simulink model "motor_model"  (R2026a)
settings: Solver=VariableStepAuto  StopTime=30  FixedStep=-1
model workspace (MAT data in the model file):
  g = 9.81
  k = 2
  r = 0.05
  t = 1800
  zs = [1.77 0.0139]
values from neighbouring files (symbols this model uses):
  amb_temp = 25    [datagenerationcode.m]
  current_gain = 1.0    (= 1)    [datagenerationcode.m]
  fault_enable = (fault_mask ~= 0)    [datagenerationcode.m]
  fault_mask = fault_masks(m)    [datagenerationcode.m]
  temp_gain = 1.0    (= 1)    [datagenerationcode.m]
  ts = 0.02    [datagenerationcode.m]
  vib_gain = 1.0    (= 1)    [datagenerationcode.m]
libraries: simulink x8, fl_lib x6, nesl_utility x3, dspfdesign x1, autolibim x1
settings Model: Creator=Onabanjo Daniel
settings SimscapeCC: SimscapeNominalValues="[{\"value\":\"1\",\"unit\":\"A\"},{\"value\":\"1\",\"unit\":\"bar\"},{\"value\":\"1\",\"unit\":\"cm^2\"},{\"value\":\"1\",\"unit\":\"cm^3/s\"},{\"value\":\"1\",\"unit\":\"kJ/kg\"},{\"value\":\"1\",\"unit\":\"kW\"},{\"value\":\"1\",\"unit\":\"l\"},{\"value\":\"1\",\"unit\":\"N\"},{\"value\":\"1\",\"unit\":\"N*m\"},{\"value\":\"1\",\"unit\":\"V\"}]"  SimscapeLogType=none  SimscapeLogDataHistory=5000.0

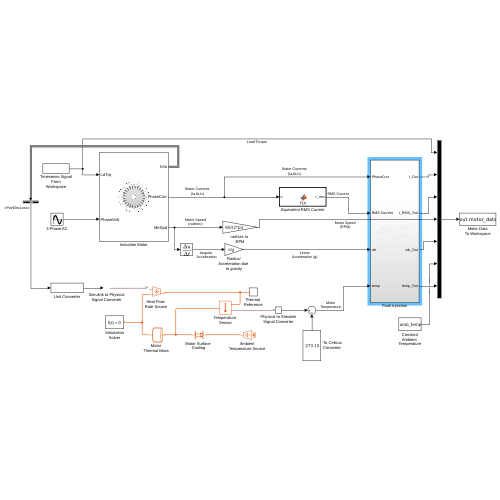
[thumbnail: Simulink's stored preview of the top-level diagram]
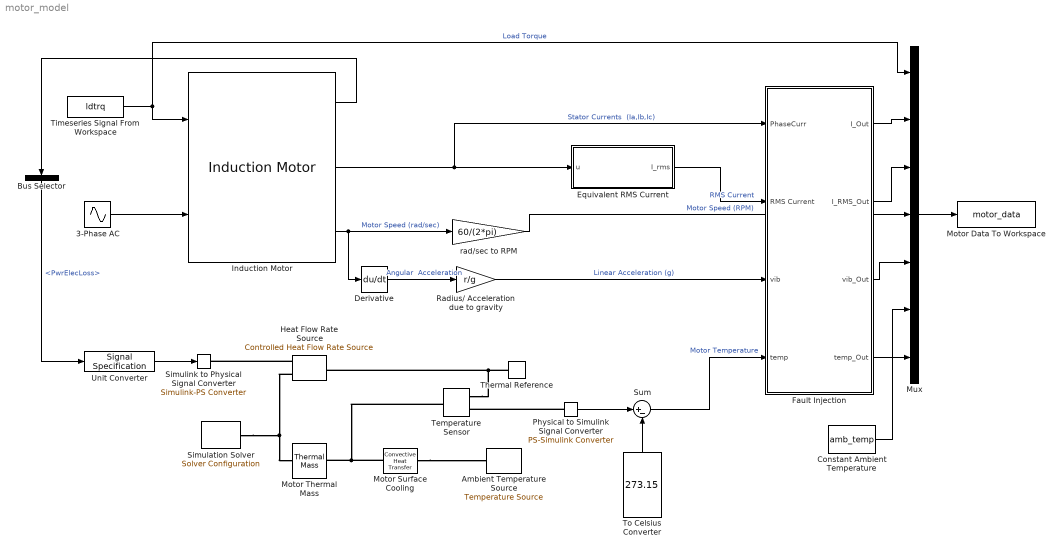
== system motor_model ==
  3-Phase AC : Sin  Amplitude=230*sqrt(2)  Frequency=2*pi*50  Phase=[0,(-2*pi/3),(-4*pi/3)]  SampleTime=0
  Ambient Temperature Source : fl_lib/Thermal/Thermal Sources/Temperature Source  temperature=298 K
  Bus Selector : BusSelector  OutputSignals=PwrInfo.PwrNotTrnsfrd.PwrElecLoss
  Constant Ambient Temperature : Constant  Value=amb_temp
  Derivative : Derivative
  Equivalent RMS Current : MATLAB Function  TreatAsAtomicUnit=on
  Fault Injection : Subsystem
  Heat Flow Rate Source : fl_lib/Thermal/Thermal Sources/Controlled Heat Flow Rate Source
  Induction Motor : autolibim/Induction Motor  sim_type=Continuous  Ts=0.001  port_config=Torque  P=2  Zs=zs  Zr="[1.34  0.0121]"  Lm=0.3687  mechanical=[0.001 0 0]  theta_init=0  omega_init=0  RefBlkName='autolibim/Induction Motor'  aMode=5
      settings: LibrarySourceBlock=mcblib/Electrical Systems/Motors/Induction Motor
  Motor Thermal Mass : fl_lib/Thermal/Thermal Elements/Thermal Mass  mass_type=foundation.enum.constant_variable.constant  mass=15 kg  sp_heat=447 J/(K*kg)  mass_min=1e-6 kg  num_ports=foundation.enum.numPorts2.two  m_specify=off  m_priority=High  m=1 kg  m_nominal_specify=off  m_nominal_value=1  m_nominal_unit=kg  T_specify=off  T_priority=High  T=300 K  T_nominal_specify=off  T_nominal_value=1  T_nominal_unit=K  Q_specify=off  Q_priority=None  Q=0 W  Q_nominal_specify=off  Q_nominal_value=1  Q_nominal_unit=W
  Motor Data To Workspace : ToWorkspace  VariableName=motor_data  SaveFormat=Timeseries  SampleTime=ts
  Motor Surface Cooling : fl_lib/Thermal/Thermal Elements/Convective Heat Transfer  thermal_type=foundation.enum.constant_variable.constant  area=1e-4 m^2  heat_tr_coeff=20 W/(K*m^2)  min_heat_tr_coeff=1e-3 W/(K*m^2)  T_specify=off  T_priority=None  T=0 K  T_nominal_specify=off  T_nominal_value=1  T_nominal_unit=K  Q_specify=off  Q_priority=None  Q=0 W  Q_nominal_specify=off  Q_nominal_value=1  Q_nominal_unit=W
  Mux : Mux  Inputs=7
  Physical to Simulink Signal Converter : nesl_utility/PS-Simulink Converter  PhysicalDomain=network_engine_domain  SubClassName=ps_output  LeftPortType=input  RightPortType=output  PseudoPeriodic=off  Frequencies=[]  VectorFormat=inherit  Unit=inherit  AffineConversion=off
  Radius/ Acceleration due to gravity : Gain  Gain=r/g
  "Simulation Solver " : nesl_utility/Solver Configuration  PhysicalDomain=network_engine_domain  SubClassName=solver  LeftPortType=input  RightPortType=generic  Tones=[]  Harmonics=[]  SimulateNoise=off  Profile=off  UseLocalSampling=off  EnableSwitchedLinearOptims=on  FrequencyDomain=off  UseCCode=off  RelTol=0.001  AbsTol=0.001  MinStep=1e-09  ToWorkspace=off  RevertToSquareIcSolve=off  NumHomotopyIterations=100  PhasorMode=off  PhasorModeNumHarmonics=1  ConsistencySolver=NEWTON_XTOL_AFTER_FTOL  CanonicalOrdering=UNORDERED  OptimizeIntermediates=UNOPTIMIZED  IndexReductionMethod=DerivativeReplacement  DoDC=off  ResidualTolerance=1e-09  ConsistencyTolSource=GLOBAL  ConsistencyAbsTol=0.001  ConsistencyRelTol=0.001  ConsistencyTolFactor=0.001  UseLocalSolver=off  LocalSolverChoice=NE_BACKWARD_EULER_ADVANCER  ResolveIndetEquations=on  FunctionEvalNumThread=1  LocalSolverSampleTime=0.001  DoFixedCost=off  MaxNonlinIter=3  MaxModeIter=2  ComputeImpulses=off  ImpulseIterations=2  LinearAlgebra=auto  LinearAlgebraNumThread=0  EquationFormulation=NE_TIME_EF  DelaysMemoryBudget=1024  AutomaticFiltering=on  FilteringTimeConstant=0.001  PartitionStorageMethod=AS_NEEDED  PartitionMemoryBudget=1024  PartitionMethod=ROBUST  MultibodyUseLocalSolver=off  MultibodyLocalSolverChoice=ODE1  MultibodyLocalSolverSampleTime=0.001
  Simulink to Physical Signal Converter : nesl_utility/Simulink-PS Converter  PhysicalDomain=network_engine_domain  SubClassName=ps_input  LeftPortType=input  RightPortType=output  PseudoPeriodic=off  Frequencies=[]  NoiseDistribution=none  NoiseParameters=[]  Unit=W  AffineConversion=off  FilteringAndDerivatives=provide  SimscapeFilterOrder=1  InputFilterTimeConstant=0.001  UdotUserProvided=0
  Sum : Sum  Inputs=|+-
  Temperature Sensor : fl_lib/Thermal/Thermal Sensors/Temperature Sensor  temperature_measure=foundation.enum.MeasurementReference.difference
  Thermal Reference : fl_lib/Thermal/Thermal Elements/Thermal Reference
  Timeseries Signal From Workspace : FromWorkspace  VariableName=ldtrq  SampleTime=ts
  To Celsius Converter : Constant  Value=273.15
  Unit Converter : SignalSpecification  Unit=W
  "rad/sec to RPM " : Gain  Gain=60/(2*pi)
  wires:
  3-Phase AC/1 -> Induction Motor/2
  Timeseries Signal From Workspace/1 -> Mux/1, Induction Motor/1  "Load Torque"
  Induction Motor/2 -> Fault Injection/1(PhaseCurr), Equivalent RMS Current/1(u)  "Stator Currents  (Ia,Ib,Ic)"
  Mux/1 -> Motor Data To Workspace/1
  Induction Motor/3 -> Derivative/1, "rad/sec to RPM "/1  "Motor Speed (rad/sec)"
  "rad/sec to RPM "/1 -> Mux/4  "Motor Speed (RPM)"
  Equivalent RMS Current/1(I_rms) -> Fault Injection/2(RMS Current)  "RMS Current"
  Derivative/1 -> Radius/ Acceleration due to gravity/1  "Angular  Acceleration"
  Radius/ Acceleration due to gravity/1 -> Fault Injection/3(vib)  "Linear Acceleration (g)"
  Bus Selector/1 -> Unit Converter/1  "<PwrElecLoss>"
  Unit Converter/1 -> Simulink to Physical Signal Converter/1
  Physical to Simulink Signal Converter/1 -> Sum/1
  Induction Motor/1 -> Bus Selector/1
  Sum/1 -> Fault Injection/4(temp)  "Motor Temperature"
  Constant Ambient Temperature/1 -> Mux/6
  To Celsius Converter/1 -> Sum/2
  Fault Injection/1(I_Out) -> Mux/2
  Fault Injection/4(temp_Out) -> Mux/7
  Fault Injection/3(vib_Out) -> Mux/5
  Fault Injection/2(I_RMS_Out) -> Mux/3
  connections:
  Heat Flow Rate Source/RConn1 -- Simulink to Physical Signal Converter/RConn1
  Heat Flow Rate Source/RConn2 -- "Simulation Solver "/RConn1 -- Motor Thermal Mass/RConn1
  Motor Surface Cooling/LConn1 -- Temperature Sensor/LConn1 -- Motor Thermal Mass/LConn1
  Physical to Simulink Signal Converter/LConn1 -- Temperature Sensor/RConn2
  Motor Surface Cooling/RConn1 -- Ambient Temperature Source/LConn1
  Thermal Reference/LConn1 -- Temperature Sensor/RConn1 -- Heat Flow Rate Source/LConn1

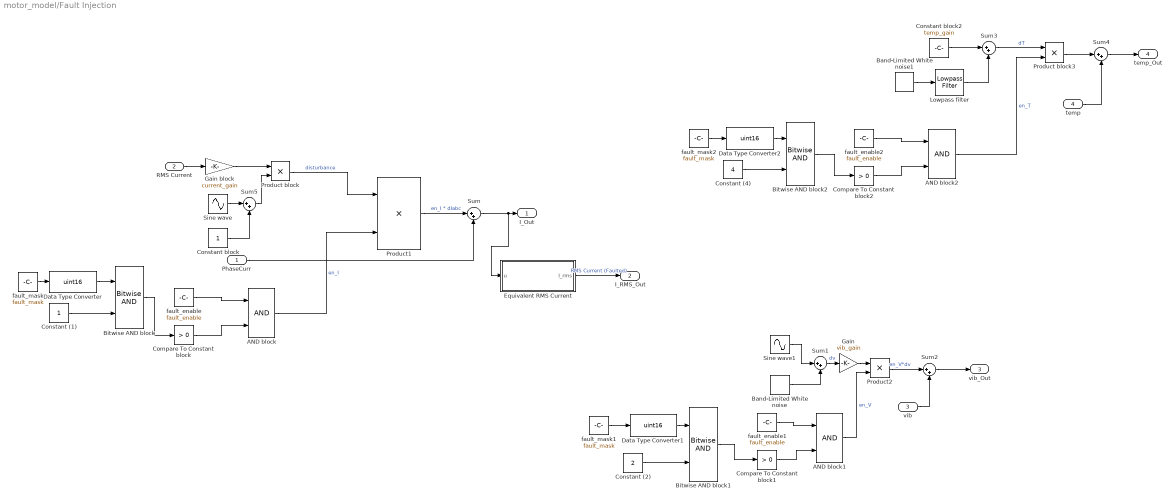
== system motor_model/Fault Injection ==
  PhaseCurr : Inport
  RMS Current : Inport  Port=2
  vib : Inport  Port=3
  temp : Inport  Port=4
  AND block : Logic  IconShape=distinctive  AllPortsSameDT=off  OutDataTypeStr=boolean
  AND block1 : Logic  IconShape=distinctive  AllPortsSameDT=off  OutDataTypeStr=boolean
  AND block2 : Logic  IconShape=distinctive  AllPortsSameDT=off  OutDataTypeStr=boolean
  Band-Limited White noise : simulink/Sources/Band-Limited White Noise  Cov=[0.1]  Ts=0.1  seed=[23341]
  Band-Limited White noise1 : simulink/Sources/Band-Limited White Noise  Cov=[0.1]  Ts=0.1  seed=[23341]
  Bitwise AND block : simulink/Logic and Bit Operations/Bitwise Operator  logicop=AND  UseBitMask=off  NumInputPorts=2  BitMask=bin2dec('11011001')  BitMaskRealWorld=Stored Integer
      settings: LibrarySourceBlock=|
      | simulink/Quick Insert/Logic and Bit
      | Operations/Bitwise AND
  Bitwise AND block1 : simulink/Logic and Bit Operations/Bitwise Operator  logicop=AND  UseBitMask=off  NumInputPorts=2  BitMask=bin2dec('11011001')  BitMaskRealWorld=Stored Integer
      settings: LibrarySourceBlock=|
      | simulink/Quick Insert/Logic and Bit
      | Operations/Bitwise AND
  Bitwise AND block2 : simulink/Logic and Bit Operations/Bitwise Operator  logicop=AND  UseBitMask=off  NumInputPorts=2  BitMask=bin2dec('11011001')  BitMaskRealWorld=Stored Integer
      settings: LibrarySourceBlock=|
      | simulink/Quick Insert/Logic and Bit
      | Operations/Bitwise AND
  Compare To Constant block : simulink/Logic and Bit Operations/Compare To Constant  relop=>  const=0  OutDataTypeStr=boolean
  Compare To Constant block1 : simulink/Logic and Bit Operations/Compare To Constant  relop=>  const=0  OutDataTypeStr=boolean
  Compare To Constant block2 : simulink/Logic and Bit Operations/Compare To Constant  relop=>  const=0  OutDataTypeStr=boolean
  Constant block : Constant
  Constant block2 : Constant  Value=temp_gain
  Constant (1) : Constant  OutDataTypeStr=uint16
  Constant (2) : Constant  Value=2  OutDataTypeStr=uint16
  Constant (4) : Constant  Value=4  OutDataTypeStr=uint16
  Data Type Converter : DataTypeConversion  OutDataTypeStr=uint16  SaturateOnIntegerOverflow=off  RndMeth=Floor
  Data Type Converter1 : DataTypeConversion  OutDataTypeStr=uint16  SaturateOnIntegerOverflow=off  RndMeth=Floor
  Data Type Converter2 : DataTypeConversion  OutDataTypeStr=uint16  SaturateOnIntegerOverflow=off  RndMeth=Floor
  Equivalent RMS Current : MATLAB Function  TreatAsAtomicUnit=on
  Gain : Gain  Gain=vib_gain
  Gain block : Gain  Gain=current_gain
  Lowpass filter : dspfdesign/Lowpass Filter  FilterType=FIR  DesignForMinimumOrder=on  FilterOrder=50  PassbandFrequency=0.3628  StopbandFrequency=0.5442  PassbandRipple=0.1  StopbandAttenuation=80  SampleRateMode=Use normalized frequency (0 to 1)  SampleRate=44100  SimulateUsing=Interpreted execution  roundingMode=Floor  coeffsDataTypeStr=fixdt(1,16)
  Product block : Product
  Product block3 : Product
  Product1 : Product
  Product2 : Product
  Sine wave : Sin  Frequency=2*pi*50  SampleTime=0
  Sine wave1 : Sin  Frequency=2*pi*100  SampleTime=0
  Sum{,1..5} (6 alike) : Sum  Inputs=|++
  fault_enable : Constant  Value=fault_enable
  fault_enable1 : Constant  Value=fault_enable
  fault_enable2 : Constant  Value=fault_enable
  fault_mask : Constant  Value=fault_mask
  fault_mask1 : Constant  Value=fault_mask
  fault_mask2 : Constant  Value=fault_mask
  I_Out : Outport
  I_RMS_Out : Outport  Port=2
  vib_Out : Outport  Port=3
  temp_Out : Outport  Port=4
  wires:
  vib/1 -> Sum2/2
  temp/1 -> Sum4/2
  RMS Current/1 -> Gain block/1
  Gain block/1 -> Product block/1
  fault_mask/1 -> Data Type Converter/1
  Bitwise AND block/1 -> Compare To Constant block/1
  AND block/1 -> Product1/2  "en_I"
  Constant (1)/1 -> Bitwise AND block/2
  Compare To Constant block1/1 -> AND block1/2
  AND block1/1 -> Product2/2  "en_V"
  fault_enable2/1 -> AND block2/1
  fault_enable1/1 -> AND block1/1
  Compare To Constant block2/1 -> AND block2/2
  Bitwise AND block2/1 -> Compare To Constant block2/1
  Constant (4)/1 -> Bitwise AND block2/2
  fault_mask2/1 -> Data Type Converter2/1
  Bitwise AND block1/1 -> Compare To Constant block1/1
  fault_mask1/1 -> Data Type Converter1/1
  Constant (2)/1 -> Bitwise AND block1/2
  AND block2/1 -> Product block3/2  "en_T"
  Compare To Constant block/1 -> AND block/2
  fault_enable/1 -> AND block/1
  Product1/1 -> Sum/1  "en_I * dIabc"
  PhaseCurr/1 -> Sum/2
  Sum/1 -> Equivalent RMS Current/1(u), I_Out/1
  Sine wave1/1 -> Sum1/1
  Band-Limited White noise/1 -> Sum1/2
  Sum1/1 -> Gain/1  "dv"
  Product2/1 -> Sum2/1  "en_V*dv"
  Sum2/1 -> vib_Out/1
  Constant block2/1 -> Sum3/1
  Lowpass filter/1 -> Sum3/2
  Sum3/1 -> Product block3/1  "dT"
  Band-Limited White noise1/1 -> Lowpass filter/1
  Product block3/1 -> Sum4/1
  Sum4/1 -> temp_Out/1
  Data Type Converter/1 -> Bitwise AND block/1
  Data Type Converter1/1 -> Bitwise AND block1/1
  Data Type Converter2/1 -> Bitwise AND block2/1
  Equivalent RMS Current/1(I_rms) -> I_RMS_Out/1  "RMS Current (Faulted)"
  Sine wave/1 -> Sum5/1
  Constant block/1 -> Sum5/2
  Sum5/1 -> Product block/2
  Product block/1 -> Product1/1  "disturbance"
  Gain/1 -> Product2/1

== matlab function motor_model/Equivalent RMS Current ==
  data: u input; I_rms output
function I_rms = fcn(u)
Ia = u(1);
Ib = u(2);
Ic = u(3);
I_rms = sqrt((Ia^2 + Ib^2 + Ic^2)/3);

== matlab function motor_model/Fault Injection/Equivalent RMS Current ==
  data: u input; I_rms output
function I_rms = fcn(u)
Ia = u(1);
Ib = u(2);
Ic = u(3);
I_rms = sqrt((Ia^2 + Ib^2 + Ic^2)/3);
